simulink library "BMSA_lib"  (Simulink 7.5)
settings: Solver=ode45  StartTime=0.0  StopTime=10.0  RelTol=1e-3
values from neighbouring files (symbols this model uses):
  pBMSA_A_ContaOpenCurr_C = Simulink.Parameter    [BMSA_par.m]
  pBMSA_s_ContStsTiout_C = Simulink.Parameter    [BMSA_par.m]
  pBMSA_s_IMeasTiout_C = Simulink.Parameter    [BMSA_par.m]
  pBMSA_s_UMeasTiout_C = Simulink.Parameter    [BMSA_par.m]
  pBMSA_V_BatUThd_C = Simulink.Parameter    [BMSA_par.m]
  pBMSA_V_ChrgUThd_C = Simulink.Parameter    [BMSA_par.m]
  pBMSA_V_UDifThd_C = Simulink.Parameter    [BMSA_par.m]
libraries: BaseOperationLib_Browser x9, simulink x1
settings Model: Creator=wuaibin  LastModifiedBy=wuaibin

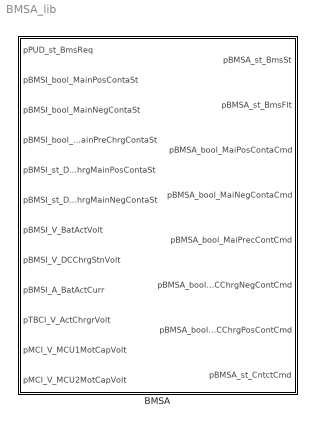
== system BMSA_lib ==
  BMSA : Subsystem  TreatAsAtomicUnit=on

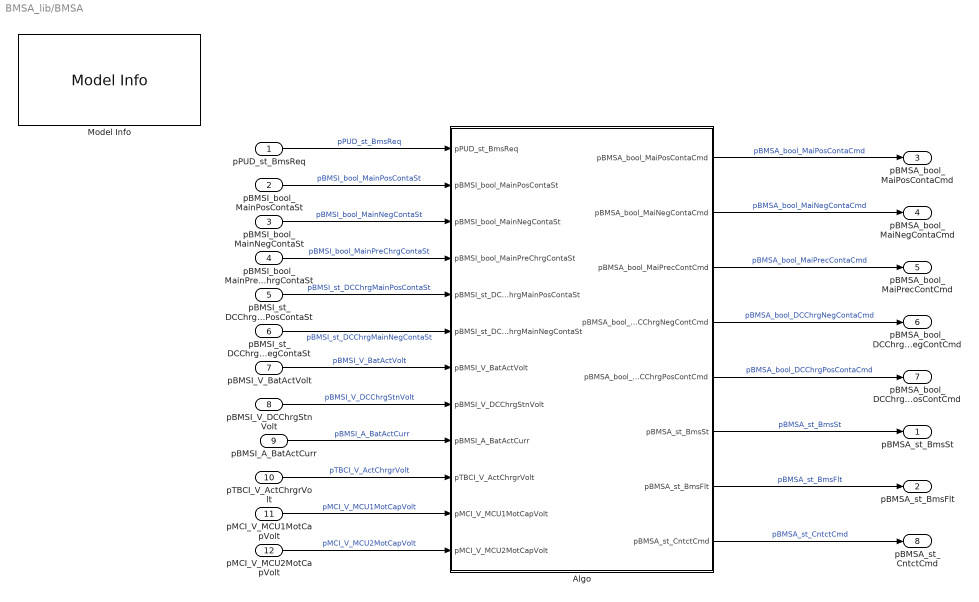
== system BMSA_lib/BMSA ==
  pPUD_st_BmsReq : Inport  OutDataType=fixdt(1, 16)  OutScaling=2^0
  pBMSI_bool_MainPosContaSt : Inport  Port=2  OutDataType=fixdt(1, 16)  OutScaling=2^0
  pBMSI_bool_MainNegContaSt : Inport  Port=3  OutDataType=fixdt(1, 16)  OutScaling=2^0
  pBMSI_bool_MainPreChrgContaSt : Inport  Port=4  OutDataType=fixdt(1, 16)  OutScaling=2^0
  pBMSI_st_DCChrgMainPosContaSt : Inport  Port=5  OutDataType=fixdt(1, 16)  OutScaling=2^0
  pBMSI_st_DCChrgMainNegContaSt : Inport  Port=6  OutDataType=fixdt(1, 16)  OutScaling=2^0
  pBMSI_V_BatActVolt : Inport  Port=7  OutDataType=fixdt(1, 16)  OutScaling=2^0
  pBMSI_V_DCChrgStnVolt : Inport  Port=8  OutDataType=fixdt(1, 16)  OutScaling=2^0
  pBMSI_A_BatActCurr : Inport  Port=9  OutDataType=fixdt(1, 16)  OutScaling=2^0
  pTBCI_V_ActChrgrVolt : Inport  Port=10  OutDataType=fixdt(1, 16)  OutScaling=2^0
  pMCI_V_MCU1MotCapVolt : Inport  Port=11  OutDataType=fixdt(1, 16)  OutScaling=2^0
  pMCI_V_MCU2MotCapVolt : Inport  Port=12  OutDataType=fixdt(1, 16)  OutScaling=2^0
  Algo : Subsystem
  Model Info : simulink/Model-Wide Utilities/Model Info  SystemSampleTime=-1  InitialBlockCM=None  BlockCM=None  Frame=on  DisplayStringWithTags=Model Info\nCreated: %<Created>\nCreator: wuaibin  HorizontalTextAlignment=Center  LeftAlignmentValue=0.5  SourceBlockDiagram=HQEV_HCU  TagMaxNumber=20
  pBMSA_st_BmsSt : Outport  OutDataType=fixdt(1, 16)  OutScaling=2^0
  pBMSA_st_BmsFlt : Outport  Port=2  OutDataType=fixdt(1, 16)  OutScaling=2^0
  pBMSA_bool_MaiPosContaCmd : Outport  Port=3  OutDataType=fixdt(1, 16)  OutScaling=2^0
  pBMSA_bool_MaiNegContaCmd : Outport  Port=4  OutDataType=fixdt(1, 16)  OutScaling=2^0
  pBMSA_bool_MaiPrecContCmd : Outport  Port=5  OutDataType=fixdt(1, 16)  OutScaling=2^0
  pBMSA_bool_DCChrgNegContCmd : Outport  Port=6  OutDataType=fixdt(1, 16)  OutScaling=2^0
  pBMSA_bool_DCChrgPosContCmd : Outport  Port=7  OutDataType=fixdt(1, 16)  OutScaling=2^0
  pBMSA_st_CntctCmd : Outport  Port=8  OutDataType=fixdt(1, 16)  OutScaling=2^0
  wires:
  pBMSI_A_BatActCurr/1 -> Algo/9(pBMSI_A_BatActCurr)  "pBMSI_A_BatActCurr"
  Algo/8(pBMSA_st_CntctCmd) -> pBMSA_st_CntctCmd/1  "pBMSA_st_CntctCmd"
  Algo/7(pBMSA_st_BmsFlt) -> pBMSA_st_BmsFlt/1  "pBMSA_st_BmsFlt"
  Algo/6(pBMSA_st_BmsSt) -> pBMSA_st_BmsSt/1  "pBMSA_st_BmsSt"
  Algo/5(pBMSA_bool_DCChrgPosContCmd) -> pBMSA_bool_DCChrgPosContCmd/1  "pBMSA_bool_DCChrgPosContaCmd"
  Algo/4(pBMSA_bool_DCChrgNegContCmd) -> pBMSA_bool_DCChrgNegContCmd/1  "pBMSA_bool_DCChrgNegContaCmd"
  Algo/3(pBMSA_bool_MaiPrecContCmd) -> pBMSA_bool_MaiPrecContCmd/1  "pBMSA_bool_MaiPrecContaCmd"
  Algo/2(pBMSA_bool_MaiNegContaCmd) -> pBMSA_bool_MaiNegContaCmd/1  "pBMSA_bool_MaiNegContaCmd"
  Algo/1(pBMSA_bool_MaiPosContaCmd) -> pBMSA_bool_MaiPosContaCmd/1  "pBMSA_bool_MaiPosContaCmd"
  pMCI_V_MCU2MotCapVolt/1 -> Algo/12(pMCI_V_MCU2MotCapVolt)  "pMCI_V_MCU2MotCapVolt"
  pMCI_V_MCU1MotCapVolt/1 -> Algo/11(pMCI_V_MCU1MotCapVolt)  "pMCI_V_MCU1MotCapVolt"
  pTBCI_V_ActChrgrVolt/1 -> Algo/10(pTBCI_V_ActChrgrVolt)  "pTBCI_V_ActChrgrVolt"
  pBMSI_V_DCChrgStnVolt/1 -> Algo/8(pBMSI_V_DCChrgStnVolt)  "pBMSI_V_DCChrgStnVolt"
  pBMSI_V_BatActVolt/1 -> Algo/7(pBMSI_V_BatActVolt)  "pBMSI_V_BatActVolt"
  pBMSI_st_DCChrgMainNegContaSt/1 -> Algo/6(pBMSI_st_DCChrgMainNegContaSt)  "pBMSI_st_DCChrgMainNegContaSt"
  pBMSI_st_DCChrgMainPosContaSt/1 -> Algo/5(pBMSI_st_DCChrgMainPosContaSt)  "pBMSI_st_DCChrgMainPosContaSt"
  pBMSI_bool_MainPreChrgContaSt/1 -> Algo/4(pBMSI_bool_MainPreChrgContaSt)  "pBMSI_bool_MainPreChrgContaSt"
  pBMSI_bool_MainNegContaSt/1 -> Algo/3(pBMSI_bool_MainNegContaSt)  "pBMSI_bool_MainNegContaSt"
  pBMSI_bool_MainPosContaSt/1 -> Algo/2(pBMSI_bool_MainPosContaSt)  "pBMSI_bool_MainPosContaSt"
  pPUD_st_BmsReq/1 -> Algo/1(pPUD_st_BmsReq)  "pPUD_st_BmsReq"

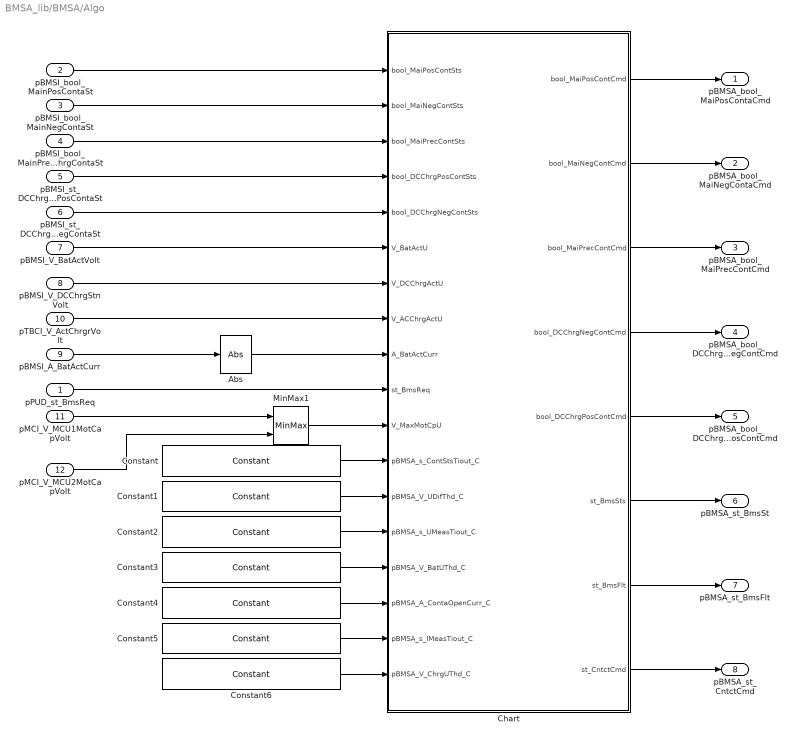
== system BMSA_lib/BMSA/Algo ==
  pPUD_st_BmsReq : Inport  OutDataType=fixdt(1, 16)  OutScaling=2^0
  pBMSI_bool_MainPosContaSt : Inport  Port=2  OutDataType=fixdt(1, 16)  OutScaling=2^0
  pBMSI_bool_MainNegContaSt : Inport  Port=3  OutDataType=fixdt(1, 16)  OutScaling=2^0
  pBMSI_bool_MainPreChrgContaSt : Inport  Port=4  OutDataType=fixdt(1, 16)  OutScaling=2^0
  pBMSI_st_DCChrgMainPosContaSt : Inport  Port=5  OutDataType=fixdt(1, 16)  OutScaling=2^0
  pBMSI_st_DCChrgMainNegContaSt : Inport  Port=6  OutDataType=fixdt(1, 16)  OutScaling=2^0
  pBMSI_V_BatActVolt : Inport  Port=7  OutDataType=fixdt(1, 16)  OutScaling=2^0
  pBMSI_V_DCChrgStnVolt : Inport  Port=8  OutDataType=fixdt(1, 16)  OutScaling=2^0
  pBMSI_A_BatActCurr : Inport  Port=9  OutDataType=fixdt(1, 16)  OutScaling=2^0
  pTBCI_V_ActChrgrVolt : Inport  Port=10  OutDataType=fixdt(1, 16)  OutScaling=2^0
  pMCI_V_MCU1MotCapVolt : Inport  Port=11  OutDataType=fixdt(1, 16)  OutScaling=2^0
  pMCI_V_MCU2MotCapVolt : Inport  Port=12  OutDataType=fixdt(1, 16)  OutScaling=2^0
  Abs : BaseOperationLib_Browser/Math Operations Changed/Abs  OutMax=[]  OutDataType=fixdt(1, 16)  OutScaling=2^0  SaturateOnIntegerOverflow=on
  Chart : Stateflow chart  TreatAsAtomicUnit=on
  Constant : BaseOperationLib_Browser/Sources&Sinks/Constant  Value=pBMSA_s_ContStsTiout_C  OutMin=[]  OutMax=[]  OutDataType=fixdt(1, 16)  ConRadixGroup=Use specified scaling  OutScaling=2^0  OutDataTypeStr=Inherit: Inherit from 'Constant value'
  Constant1 : BaseOperationLib_Browser/Sources&Sinks/Constant  Value=pBMSA_V_UDifThd_C  OutMin=[]  OutMax=[]  OutDataType=fixdt(1, 16)  ConRadixGroup=Use specified scaling  OutScaling=2^0  OutDataTypeStr=Inherit: Inherit from 'Constant value'
  Constant2 : BaseOperationLib_Browser/Sources&Sinks/Constant  Value=pBMSA_s_UMeasTiout_C  OutMin=[]  OutMax=[]  OutDataType=fixdt(1, 16)  ConRadixGroup=Use specified scaling  OutScaling=2^0  OutDataTypeStr=Inherit: Inherit from 'Constant value'
  Constant3 : BaseOperationLib_Browser/Sources&Sinks/Constant  Value=pBMSA_V_BatUThd_C  OutMin=[]  OutMax=[]  OutDataType=fixdt(1, 16)  ConRadixGroup=Use specified scaling  OutScaling=2^0  OutDataTypeStr=Inherit: Inherit from 'Constant value'
  Constant4 : BaseOperationLib_Browser/Sources&Sinks/Constant  Value=pBMSA_A_ContaOpenCurr_C  OutMin=[]  OutMax=[]  OutDataType=fixdt(1, 16)  ConRadixGroup=Use specified scaling  OutScaling=2^0  OutDataTypeStr=Inherit: Inherit from 'Constant value'
  Constant5 : BaseOperationLib_Browser/Sources&Sinks/Constant  Value=pBMSA_s_IMeasTiout_C  OutMin=[]  OutMax=[]  OutDataType=fixdt(1, 16)  ConRadixGroup=Use specified scaling  OutScaling=2^0  OutDataTypeStr=Inherit: Inherit from 'Constant value'
  Constant6 : BaseOperationLib_Browser/Sources&Sinks/Constant  Value=pBMSA_V_ChrgUThd_C  OutMin=[]  OutMax=[]  OutDataType=fixdt(1, 16)  ConRadixGroup=Use specified scaling  OutScaling=2^0  OutDataTypeStr=Inherit: Inherit from 'Constant value'
  MinMax1 : BaseOperationLib_Browser/Math Operations Changed/MinMax  Function=max  Inputs=2  InputSameDT=on  OutMin=[]  OutMax=[]  OutDataType=fixdt(1, 16)  OutScaling=2^0  SaturateOnIntegerOverflow=on
  pBMSA_bool_MaiPosContaCmd : Outport  OutDataType=fixdt(1, 16)  OutScaling=2^0
  pBMSA_bool_MaiNegContaCmd : Outport  Port=2  OutDataType=fixdt(1, 16)  OutScaling=2^0
  pBMSA_bool_MaiPrecContCmd : Outport  Port=3  OutDataType=fixdt(1, 16)  OutScaling=2^0
  pBMSA_bool_DCChrgNegContCmd : Outport  Port=4  OutDataType=fixdt(1, 16)  OutScaling=2^0
  pBMSA_bool_DCChrgPosContCmd : Outport  Port=5  OutDataType=fixdt(1, 16)  OutScaling=2^0
  pBMSA_st_BmsSt : Outport  Port=6  OutDataType=fixdt(1, 16)  OutScaling=2^0
  pBMSA_st_BmsFlt : Outport  Port=7  OutDataType=fixdt(1, 16)  OutScaling=2^0
  pBMSA_st_CntctCmd : Outport  Port=8  OutDataType=fixdt(1, 16)  OutScaling=2^0
  wires:
  Constant5/1 -> Chart/17(pBMSA_s_IMeasTiout_C)
  Constant4/1 -> Chart/16(pBMSA_A_ContaOpenCurr_C)
  Constant3/1 -> Chart/15(pBMSA_V_BatUThd_C)
  Constant2/1 -> Chart/14(pBMSA_s_UMeasTiout_C)
  Constant1/1 -> Chart/13(pBMSA_V_UDifThd_C)
  Constant/1 -> Chart/12(pBMSA_s_ContStsTiout_C)
  Abs/1 -> Chart/9(A_BatActCurr)
  pBMSI_A_BatActCurr/1 -> Abs/1
  MinMax1/1 -> Chart/11(V_MaxMotCpU)
  Chart/8(st_CntctCmd) -> pBMSA_st_CntctCmd/1
  pBMSI_V_DCChrgStnVolt/1 -> Chart/7(V_DCChrgActU)
  pTBCI_V_ActChrgrVolt/1 -> Chart/8(V_ACChrgActU)
  Chart/5(bool_DCChrgPosContCmd) -> pBMSA_bool_DCChrgPosContCmd/1
  Chart/4(bool_DCChrgNegContCmd) -> pBMSA_bool_DCChrgNegContCmd/1
  pBMSI_st_DCChrgMainNegContaSt/1 -> Chart/5(bool_DCChrgNegContSts)
  pBMSI_st_DCChrgMainPosContaSt/1 -> Chart/4(bool_DCChrgPosContSts)
  Chart/1(bool_MaiPosContCmd) -> pBMSA_bool_MaiPosContaCmd/1
  Chart/2(bool_MaiNegContCmd) -> pBMSA_bool_MaiNegContaCmd/1
  Chart/3(bool_MaiPrecContCmd) -> pBMSA_bool_MaiPrecContCmd/1
  pPUD_st_BmsReq/1 -> Chart/10(st_BmsReq)
  pBMSI_bool_MainPosContaSt/1 -> Chart/1(bool_MaiPosContSts)
  pBMSI_bool_MainNegContaSt/1 -> Chart/2(bool_MaiNegContSts)
  pBMSI_bool_MainPreChrgContaSt/1 -> Chart/3(bool_MaiPrecContSts)
  Chart/6(st_BmsSts) -> pBMSA_st_BmsSt/1
  pBMSI_V_BatActVolt/1 -> Chart/6(V_BatActU)
  Chart/7(st_BmsFlt) -> pBMSA_st_BmsFlt/1
  pMCI_V_MCU1MotCapVolt/1 -> MinMax1/1
  pMCI_V_MCU2MotCapVolt/1 -> MinMax1/2
  Constant6/1 -> Chart/18(pBMSA_V_ChrgUThd_C)

== stateflow chart BMSA/Algo/Chart ==
  state Normal
    state HV_OFF
      entry:
      st_CntctCmd = CntctStsTyp.CNT_HVOFF;
      state OpenDCChrgPosContactor
        entry:
        bool_DCChrgPosContCmd = false;
      state OpenDCChrgNegContactor
        entry:
        bool_DCChrgNegContCmd = false;
      state OpenMainPositive
        entry:
        bool_MaiPosContCmd = false;
      state NormWarning
        entry:
        bool_DCChrgPosContCmd = false;
        bool_DCChrgNegContCmd = false;
        bool_MaiPosContCmd = false;
        bool_MaiPrecContCmd = false;
        bool_MaiNegContCmd = false;
        st_BmsFlt = ERRFltTypBMSAlgo.HV_OFF_WARN;
        state Error
          en:
          st_BmsSts = BMSStsTyp.BMS_HVOFF_ERR;
        (default) -> Normal.HV_OFF.NormWarning.Error
      state OpenMainNegative
        entry:
        bool_MaiNegContCmd = false;
      state OpenPrecharge
        entry:
        bool_MaiPrecContCmd = false;
      state NormHVisOff
        entry:
        st_BmsSts = BMSStsTyp.BMS_HVOFF_OK;
      state CurrMeasurement
      OpenDCChrgPosContactor -> OpenDCChrgNegContactor [order 2] : [bool_DCChrgPosContSts == false]
      OpenDCChrgPosContactor -> (junction 80) [order 1] : after(pBMSA_s_ContStsTiout_C,sec)
      CurrMeasurement -> OpenDCChrgPosContactor : [A_BatActCurr < pBMSA_A_ContaOpenCurr_C || ...
          | after(pBMSA_s_IMeasTiout_C,sec)]
      (junction 80) -> (junction 95)
      OpenDCChrgNegContactor -> (junction 95) [order 1] : after(pBMSA_s_ContStsTiout_C,sec)
      (junction 82) -> NormWarning
      OpenMainNegative -> (junction 82) [order 1] : after(pBMSA_s_ContStsTiout_C,sec)
      (junction 95) -> (junction 84)
      (junction 81) -> (junction 82)
      Normal.HV_OFF.OpenPrecharge -> (junction 81) [order 1] : after(pBMSA_s_ContStsTiout_C,sec)
      OpenMainPositive -> (junction 84) [order 1] : after(pBMSA_s_ContStsTiout_C,sec)
      (junction 84) -> (junction 81)
      OpenMainPositive -> Normal.HV_OFF.OpenPrecharge [order 2] : [bool_MaiPosContSts == false]
      Normal.HV_OFF.OpenPrecharge -> OpenMainNegative [order 2] : [bool_MaiPrecContSts == false]
      OpenMainNegative -> NormHVisOff [order 2] : [bool_MaiNegContSts == false]
      OpenDCChrgNegContactor -> OpenMainPositive [order 2] : [bool_DCChrgNegContSts == false]
      (default) -> CurrMeasurement
      NormWarning -> NormHVisOff : [bool_DCChrgPosContSts == false && ...
          | bool_DCChrgNegContSts == false && ...
          | bool_MaiPosContSts == false && ...
          | bool_MaiPrecContSts == false && ...
          | bool_MaiNegContSts == false]
    state DCHeatON
      entry:
      st_CntctCmd = CntctStsTyp.CNT_DCHeatON;
      state DCChrgONSequenceDone
        entry:
        st_BmsSts = BMSStsTyp.BMS_DCHeatOn;
      state HV_Error
        entry:
        st_BmsSts = BMSStsTyp.BMS_DCHeatOn_ERR;
      state OpenPrecharge
        entry:
        bool_MaiPrecContCmd = false;
      state ClosePrecharge
        entry:
        bool_MaiPrecContCmd = true;
      state CloseMainPositive
        entry:
        bool_MaiPosContCmd = true;
      state MCUVoltageMeasurement
      state CloseDCChrgPosContactor
        entry:
        bool_DCChrgPosContCmd = true;
      state CloseDCChrgNegContactor
        entry:
        bool_DCChrgNegContCmd = true;
      (junction 69) -> Normal.DCHeatON.HV_Error : {st_BmsFlt = ERRFltTypBMSAlgo.HV_ON_FLT;}
      Normal.DCHeatON.OpenPrecharge -> Normal.DCHeatON.DCChrgONSequenceDone [order 1] : [bool_MaiPrecContSts == false]
      Normal.DCHeatON.OpenPrecharge -> (junction 69) [order 2] : after(pBMSA_s_ContStsTiout_C,sec)
      Normal.DCHeatON.CloseMainPositive -> Normal.DCHeatON.OpenPrecharge [order 2] : [bool_MaiPosContSts == true]
      (junction 71) -> (junction 69)
      Normal.DCHeatON.CloseMainPositive -> (junction 71) [order 1] : after(pBMSA_s_ContStsTiout_C,sec)
      Normal.DCHeatON.MCUVoltageMeasurement -> Normal.DCHeatON.CloseMainPositive [order 2] : [abs(V_DCChrgActU-V_MaxMotCpU) <= pBMSA_V_UDifThd_C && ...
          | V_MaxMotCpU >= pBMSA_V_ChrgUThd_C ]
      (junction 70) -> (junction 71)
      Normal.DCHeatON.MCUVoltageMeasurement -> (junction 70) [order 1] : after(pBMSA_s_UMeasTiout_C,sec)
      Normal.DCHeatON.ClosePrecharge -> Normal.DCHeatON.MCUVoltageMeasurement [order 2] : [bool_MaiPrecContSts == true]
      (junction 72) -> (junction 70)
      Normal.DCHeatON.ClosePrecharge -> (junction 72) [order 1] : after(pBMSA_s_ContStsTiout_C,sec)
      Normal.DCHeatON.CloseDCChrgPosContactor -> Normal.DCHeatON.ClosePrecharge [order 1] : [bool_DCChrgPosContSts == true]
      (junction 65) -> (junction 72)
      Normal.DCHeatON.CloseDCChrgPosContactor -> (junction 65) [order 2] : after(pBMSA_s_ContStsTiout_C,sec)
      Normal.DCHeatON.CloseDCChrgNegContactor -> Normal.DCHeatON.CloseDCChrgPosContactor [order 1] : [bool_DCChrgNegContSts == true]
      (junction 68) -> (junction 65)
      Normal.DCHeatON.CloseDCChrgNegContactor -> (junction 68) [order 2] : after(pBMSA_s_ContStsTiout_C,sec)
      (default) -> Normal.DCHeatON.CloseDCChrgNegContactor
    state ACHeatON
      entry:
      st_CntctCmd = CntctStsTyp.CNT_ACHeatON;
      state HV_Error
        entry:
        st_BmsSts = BMSStsTyp.BMS_ACHeatOn_ERR;
      state MCUVoltageMeasurement
      state ACHeatONSequenceDone
        entry:
        st_BmsSts = BMSStsTyp.BMS_ACHeatOn;
      Normal.ACHeatON.MCUVoltageMeasurement -> (junction 73) [order 2] : after(pBMSA_s_UMeasTiout_C,sec)
      Normal.ACHeatON.MCUVoltageMeasurement -> ACHeatONSequenceDone [order 1] : [abs(V_ACChrgActU-V_MaxMotCpU) <= pBMSA_V_UDifThd_C&& ...
          | V_MaxMotCpU >= pBMSA_V_ChrgUThd_C ]
      (junction 73) -> Normal.ACHeatON.HV_Error : {st_BmsFlt = ERRFltTypBMSAlgo.HV_ON_FLT;}
      (default) -> Normal.ACHeatON.MCUVoltageMeasurement
    state HV_ON
      entry:
      st_CntctCmd = CntctStsTyp.CNT_HVON;
      state CheckDCChrgContactorStates
        entry:
        bool_DCChrgPosContCmd = false;
        bool_DCChrgNegContCmd = false;
      state HVONSequenceDone
        entry:
        st_BmsSts = BMSStsTyp.BMS_HVOn;
      state OpenPrecharge
        entry:
        bool_MaiPrecContCmd = false;
      state HV_Error
        entry:
        st_BmsSts = BMSStsTyp.BMS_HVOn_ERR;
      state CloseMainPositive
        entry:
        bool_MaiPosContCmd = true;
      state MCUVoltageMeasurement
      state ClosePrecharge
        entry:
        bool_MaiPrecContCmd = true;
      state CloseMainNegative
        entry:
        bool_MaiNegContCmd = true;
      state CheckContactorStates
        Normal.HV_ON.CheckContactorStates -> Normal.HV_ON.CheckContactorStates [order 1] : [bool_MaiPosContSts == true && bool_MaiNegContSts == false]
            | {bool_MaiPosContCmd = false;}
      (default) -> CheckDCChrgContactorStates
      Normal.HV_ON.CloseMainNegative -> (junction 93) [order 1] : after(pBMSA_s_ContStsTiout_C,sec)
      Normal.HV_ON.OpenPrecharge -> HVONSequenceDone [order 2] : [bool_MaiPrecContSts == false]
      Normal.HV_ON.OpenPrecharge -> Normal.HV_ON.HV_Error [order 1] : [after(pBMSA_s_ContStsTiout_C,sec)]
          | {st_BmsFlt = ERRFltTypBMSAlgo.OPEN_PREC_CONT_WARN;}
      Normal.HV_ON.CloseMainPositive -> Normal.HV_ON.OpenPrecharge [order 2] : [bool_MaiPosContSts == true]
      (junction 90) -> Normal.HV_ON.HV_Error : {st_BmsFlt = ERRFltTypBMSAlgo.HV_ON_FLT;}
      Normal.HV_ON.CloseMainPositive -> (junction 90) [order 1] : after(pBMSA_s_ContStsTiout_C,sec)
      Normal.HV_ON.MCUVoltageMeasurement -> Normal.HV_ON.CloseMainPositive [order 2] : [abs(V_BatActU-V_MaxMotCpU) <= pBMSA_V_UDifThd_C && ...
          | V_MaxMotCpU >= pBMSA_V_BatUThd_C]
      (junction 91) -> (junction 90)
      Normal.HV_ON.MCUVoltageMeasurement -> (junction 91) [order 1] : after(pBMSA_s_UMeasTiout_C,sec)
      Normal.HV_ON.ClosePrecharge -> Normal.HV_ON.MCUVoltageMeasurement [order 2] : [bool_MaiPrecContSts == true || ...
          | bool_MaiPosContSts == true]
      (junction 92) -> (junction 91)
      Normal.HV_ON.ClosePrecharge -> (junction 92) [order 1] : after(pBMSA_s_ContStsTiout_C,sec)
      Normal.HV_ON.CloseMainNegative -> Normal.HV_ON.ClosePrecharge [order 2] : [bool_MaiNegContSts == true]
      (junction 93) -> (junction 92)
      Normal.HV_ON.CheckContactorStates -> Normal.HV_ON.CloseMainNegative [order 2] : [bool_MaiPosContSts == false || ...
          | bool_MaiNegContSts == true && bool_MaiPosContSts == true]
      (junction 94) -> (junction 93)
      Normal.HV_ON.CheckContactorStates -> (junction 94) [order 1] : after(pBMSA_s_ContStsTiout_C,sec)
      (junction 96) -> (junction 94)
      CheckDCChrgContactorStates -> Normal.HV_ON.CheckContactorStates [order 2] : [bool_DCChrgPosContSts == false && ...
          | bool_DCChrgNegContSts == false]
      CheckDCChrgContactorStates -> (junction 96) [order 1] : after(pBMSA_s_ContStsTiout_C,sec)
    state DCChrgON
      entry:
      st_CntctCmd = CntctStsTyp.CNT_DCChrgON;
      state CloseMainNegative
        entry:
        bool_MaiNegContCmd = true;
      state DCChrgONSequenceDone
        entry:
        st_BmsSts = BMSStsTyp.BMS_DCChrgOn;
      state HV_Error
        entry:
        st_BmsSts = BMSStsTyp.BMS_DCChrgOn_ERR;
      state CheckContactorStates
        Normal.DCChrgON.CheckContactorStates -> Normal.DCChrgON.CheckContactorStates [order 1] : [bool_MaiPosContSts == true && bool_MaiNegContSts == false]
            | {bool_MaiPosContCmd = false;}
      state ClosePrecharge
        entry:
        bool_MaiPrecContCmd = true;
      state MCUVoltageMeasurement
      state CloseMainPositive
        entry:
        bool_MaiPosContCmd = true;
      state CloseDCChrgPosContactor
        entry:
        bool_DCChrgPosContCmd = true;
      state CloseDCChrgNegContactor
        entry:
        bool_DCChrgNegContCmd = true;
      state OpenPrecharge
        entry:
        bool_MaiPrecContCmd = false;
      (default) -> Normal.DCChrgON.CheckContactorStates
      Normal.DCChrgON.CheckContactorStates -> (junction 66) [order 1] : after(pBMSA_s_ContStsTiout_C,sec)
      (junction 66) -> (junction 67)
      Normal.DCChrgON.CheckContactorStates -> Normal.DCChrgON.CloseMainNegative [order 2] : [bool_MaiPosContSts == false || ...
          |  bool_MaiNegContSts == true]
      Normal.DCChrgON.CloseMainNegative -> (junction 67) [order 1] : after(pBMSA_s_ContStsTiout_C,sec)
      (junction 67) -> (junction 74)
      Normal.DCChrgON.CloseMainNegative -> Normal.DCChrgON.ClosePrecharge [order 2] : [bool_MaiNegContSts == true]
      Normal.DCChrgON.ClosePrecharge -> (junction 74) [order 1] : after(pBMSA_s_ContStsTiout_C,sec)
      (junction 74) -> (junction 75)
      Normal.DCChrgON.ClosePrecharge -> Normal.DCChrgON.MCUVoltageMeasurement [order 2] : [bool_MaiPrecContSts == true || ...
          |  bool_MaiPosContSts == true]
      Normal.DCChrgON.MCUVoltageMeasurement -> (junction 75) [order 1] : after(pBMSA_s_UMeasTiout_C,sec)
      (junction 75) -> (junction 76)
      Normal.DCChrgON.MCUVoltageMeasurement -> Normal.DCChrgON.CloseMainPositive [order 2] : [abs(V_BatActU-V_MaxMotCpU) <= pBMSA_V_UDifThd_C && ...
          | V_MaxMotCpU >= pBMSA_V_BatUThd_C]
      Normal.DCChrgON.CloseMainPositive -> (junction 76) [order 1] : after(pBMSA_s_ContStsTiout_C,sec)
      (junction 76) -> (junction 77)
      Normal.DCChrgON.CloseMainPositive -> Normal.DCChrgON.OpenPrecharge [order 2] : [bool_MaiPosContSts == true]
      Normal.DCChrgON.CloseDCChrgPosContactor -> (junction 78) [order 2] : after(pBMSA_s_ContStsTiout_C,sec)
      (junction 77) -> (junction 78)
      Normal.DCChrgON.CloseDCChrgPosContactor -> Normal.DCChrgON.CloseDCChrgNegContactor [order 1] : [bool_DCChrgPosContSts == true]
      Normal.DCChrgON.CloseDCChrgNegContactor -> (junction 79) [order 1] : after(pBMSA_s_ContStsTiout_C,sec)
      (junction 78) -> (junction 79)
      Normal.DCChrgON.CloseDCChrgNegContactor -> Normal.DCChrgON.DCChrgONSequenceDone [order 2] : [bool_DCChrgNegContSts == true]
      Normal.DCChrgON.OpenPrecharge -> (junction 77) [order 2] : after(pBMSA_s_ContStsTiout_C,sec)
      Normal.DCChrgON.OpenPrecharge -> Normal.DCChrgON.CloseDCChrgPosContactor [order 1] : [bool_MaiPrecContSts == false]
      (junction 79) -> Normal.DCChrgON.HV_Error : {st_BmsFlt = ERRFltTypBMSAlgo.HV_ON_FLT;}
    state INIT
      entry:
      st_CntctCmd = CntctStsTyp.CNT_INIT;
      state OpenAllContactors
        entry:
        bool_DCChrgPosContCmd = false;
        bool_DCChrgNegContCmd = false;
        bool_MaiPosContCmd = false;
        bool_MaiPrecContCmd = false;
        bool_MaiNegContCmd = false;
      (default) -> Normal.INIT.OpenAllContactors
    state ACChrgON
      entry:
      st_CntctCmd = CntctStsTyp.CNT_ACChrgON;
      state ACChrgONSequenceDone
        entry:
        st_BmsSts = BMSStsTyp.BMS_ACChrgOn;
      state CheckDCChrgPosContactorStates
        entry:
        bool_DCChrgPosContCmd = false;
        bool_DCChrgNegContCmd = false;
      state CheckContactorStates
        Normal.ACChrgON.CheckContactorStates -> Normal.ACChrgON.CheckContactorStates [order 1] : [bool_MaiPosContSts == true && bool_MaiNegContSts == false]
            | {bool_MaiPosContCmd = false;}
      state CloseMainNegative
        entry:
        bool_MaiNegContCmd = true;
      state ClosePrecharge
        entry:
        bool_MaiPrecContCmd = true;
      state MCUVoltageMeasurement
      state CloseMainPositive
        entry:
        bool_MaiPosContCmd = true;
      state ACChrg_Error
        entry:
        st_BmsSts = BMSStsTyp.BMS_ACChrgOn_ERR;
      state OpenPrecharge
        entry:
        bool_MaiPrecContCmd = false;
      (junction 87) -> (junction 88)
      (default) -> CheckDCChrgPosContactorStates
      CheckDCChrgPosContactorStates -> (junction 83) [order 1] : after(pBMSA_s_ContStsTiout_C,sec)
      (junction 83) -> (junction 85)
      CheckDCChrgPosContactorStates -> Normal.ACChrgON.CheckContactorStates [order 2] : [bool_DCChrgPosContSts == false && ...
          | bool_DCChrgNegContSts == false]
      Normal.ACChrgON.CheckContactorStates -> (junction 85) [order 1] : after(pBMSA_s_ContStsTiout_C,sec)
      (junction 85) -> (junction 86)
      Normal.ACChrgON.CheckContactorStates -> Normal.ACChrgON.CloseMainNegative [order 2] : [bool_MaiPosContSts == false || ...
          |  bool_MaiNegContSts == true]
      Normal.ACChrgON.CloseMainNegative -> (junction 86) [order 1] : after(pBMSA_s_ContStsTiout_C,sec)
      (junction 86) -> (junction 87)
      Normal.ACChrgON.CloseMainNegative -> Normal.ACChrgON.ClosePrecharge [order 2] : [bool_MaiNegContSts == true]
      Normal.ACChrgON.ClosePrecharge -> (junction 87) [order 1] : after(pBMSA_s_ContStsTiout_C,sec)
      Normal.ACChrgON.ClosePrecharge -> Normal.ACChrgON.MCUVoltageMeasurement [order 2] : [bool_MaiPrecContSts == true || ...
          |  bool_MaiPosContSts == true]
      Normal.ACChrgON.MCUVoltageMeasurement -> (junction 88) [order 1] : after(pBMSA_s_UMeasTiout_C,sec)
      (junction 88) -> (junction 89)
      Normal.ACChrgON.MCUVoltageMeasurement -> Normal.ACChrgON.CloseMainPositive [order 2] : [abs(V_BatActU-V_MaxMotCpU) <= pBMSA_V_UDifThd_C && ...
          | V_MaxMotCpU >= pBMSA_V_BatUThd_C ]
      Normal.ACChrgON.CloseMainPositive -> (junction 89) [order 1] : after(pBMSA_s_ContStsTiout_C,sec)
      (junction 89) -> ACChrg_Error : {st_BmsFlt = ERRFltTypBMSAlgo.HV_ON_FLT;}
      Normal.ACChrgON.CloseMainPositive -> Normal.ACChrgON.OpenPrecharge [order 2] : [bool_MaiPosContSts == true]
      Normal.ACChrgON.OpenPrecharge -> ACChrgONSequenceDone [order 1] : [bool_MaiPrecContSts == false]
      Normal.ACChrgON.OpenPrecharge -> ACChrg_Error [order 2] : [after(pBMSA_s_ContStsTiout_C,sec)]
          | {st_BmsFlt = ERRFltTypBMSAlgo.OPEN_PREC_CONT_WARN;}
    HV_OFF -> DCChrgON [order 3] : [st_BmsReq == BMSCmdTyp.BMS_CMD_DCChrgOn]
    ACHeatON -> HV_OFF : [st_BmsReq ~= BMSCmdTyp.BMS_CMD_ACHeatOn]
    (default) -> INIT
    INIT -> DCChrgON [order 4] : [st_BmsReq == BMSCmdTyp.BMS_CMD_DCChrgOn]
    INIT -> ACChrgON [order 6] : [st_BmsReq == BMSCmdTyp.BMS_CMD_ACChrgOn]
    HV_OFF -> ACChrgON [order 4] : [st_BmsReq == BMSCmdTyp.BMS_CMD_ACChrgOn]
    HV_OFF -> ACHeatON [order 2] : [st_BmsReq == BMSCmdTyp.BMS_CMD_ACHeatOn]
    HV_OFF -> DCHeatON [order 1] : [st_BmsReq == BMSCmdTyp.BMS_CMD_DCHeatOn]
    INIT -> HV_OFF [order 5] : [st_BmsReq == BMSCmdTyp.BMS_CMD_HVOFF]
    DCChrgON -> HV_OFF : [st_BmsReq ~= BMSCmdTyp.BMS_CMD_DCChrgOn]
    HV_OFF -> HV_ON [order 5] : [st_BmsReq == BMSCmdTyp.BMS_CMD_HVOn]
    INIT -> HV_ON [order 2] : [st_BmsReq == BMSCmdTyp.BMS_CMD_HVOn]
    DCHeatON -> HV_OFF : [st_BmsReq ~= BMSCmdTyp.BMS_CMD_DCHeatOn]
    INIT -> DCHeatON [order 3] : [st_BmsReq == BMSCmdTyp.BMS_CMD_DCHeatOn]
    ACChrgON -> HV_OFF : [st_BmsReq ~= BMSCmdTyp.BMS_CMD_ACChrgOn]
    INIT -> ACHeatON [order 1] : [st_BmsReq == BMSCmdTyp.BMS_CMD_ACHeatOn]
    HV_ON -> HV_OFF : [st_BmsReq ~= BMSCmdTyp.BMS_CMD_HVOn]
  state EmgHV_OFF
    entry:
    st_CntctCmd = CntctStsTyp.CNT_EmgHVOFF;
    state OpenAllContactors
      entry:
      bool_DCChrgPosContCmd = false;
      bool_DCChrgNegContCmd = false;
      bool_MaiPosContCmd = false;
      bool_MaiPrecContCmd = false;
      bool_MaiNegContCmd = false;
    state Warning
      entry:
      st_BmsFlt = ERRFltTypBMSAlgo.HV_OFF_WARN;
      state Error
        en:
        st_BmsSts = BMSStsTyp.BMS_EmgHVOFF_ERR;
      (default) -> EmgHV_OFF.Warning.Error
      EmgHV_OFF.Warning.Error -> EmgHV_OFF.Warning.Error : [bool_DCChrgPosContSts == false && ...
          | bool_DCChrgNegContSts == false && ...
          | bool_MaiPosContSts == false && ...
          | bool_MaiPrecContSts == false && ...
          | bool_MaiNegContSts == false]
          | {st_BmsSts = BMSStsTyp.BMS_EmgHVOFF_OK;}
    state HVisOff
      entry:
      st_BmsSts = BMSStsTyp.BMS_EmgHVOFF_OK;
    EmgHV_OFF.OpenAllContactors -> HVisOff [order 2] : [bool_DCChrgPosContSts == false && ...
        | bool_DCChrgNegContSts == false && ...
        | bool_MaiNegContSts == false && ...
        | bool_MaiPrecContSts == false && ...
        | bool_MaiNegContSts == false]
    (default) -> EmgHV_OFF.OpenAllContactors
    EmgHV_OFF.OpenAllContactors -> Warning [order 1] : after(pBMSA_s_ContStsTiout_C,sec)
    Warning -> HVisOff : [bool_DCChrgPosContSts == false && ...
        | bool_DCChrgNegContSts == false && ...
        | bool_MaiNegContSts == false && ...
        | bool_MaiPrecContSts == false && ...
        | bool_MaiNegContSts == false]
  (default) -> Normal
  Normal -> EmgHV_OFF : [st_BmsReq == BMSCmdTyp.BMS_CMD_EmgHVOFF]
  data: bool_MaiPosContCmd output boolean; bool_MaiNegContCmd output boolean; bool_MaiPrecContCmd output boolean; bool_MaiPosContSts input double; bool_MaiNegContSts input double; bool_MaiPrecContSts input double; bool_DCChrgPosContSts input double; bool_DCChrgNegContSts input double; V_BatActU input double; V_DCChrgActU input double; V_ACChrgActU input double; A_BatActCurr input double; st_BmsReq input double; V_MaxMotCpU input double; pBMSA_s_ContStsTiout_C input double; pBMSA_V_UDifThd_C input double; pBMSA_s_UMeasTiout_C input double; bool_DCChrgNegContCmd output boolean; bool_DCChrgPosContCmd output boolean; st_BmsSts output uint8; st_BmsFlt output uint8; pBMSA_V_BatUThd_C input double; st_CntctCmd output uint8; pBMSA_A_ContaOpenCurr_C input double; pBMSA_s_IMeasTiout_C input double; pBMSA_V_ChrgUThd_C input double
